simulink model "simz"  (R2018b)
settings: Solver=VariableStepAuto  StartTime=0.0  StopTime=500  RelTol=1e-3
undefined symbols (not defined in the file or in its folder): fswParams, MEKF_lib, test_lib
libraries: dspmtrx3 x2, sharedutil x2, aerolibutil x2, MEKF_Conversion_lib x1, Environment_lib x1, MEKF_lib x1, Sensors_Lib x1, satelliteDynamics_lib x1
settings Model: Creator=kylle  LastModifiedBy=kylle
settings DataIOCC: SaveFormat=StructureWithTime
settings DebuggingCC: SignalResolutionControl=None

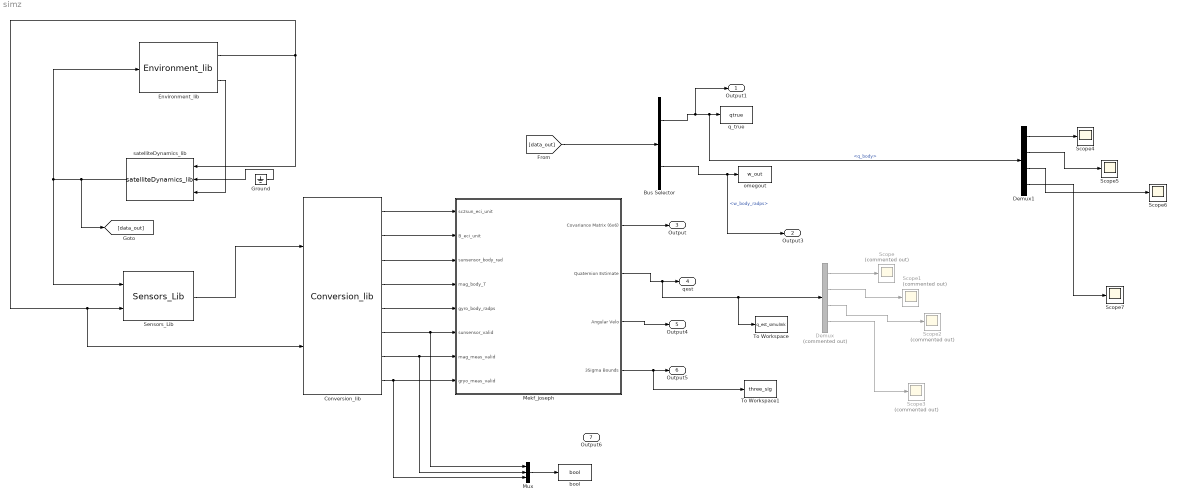
== system simz ==
  Bus Selector : BusSelector  OutputSignals=q_body,w_body_radps
  Conversion_lib : MEKF_Conversion_lib/Conversion_lib  SystemSampleTime=-1
  Demux : Demux  Commented=on
  Demux1 : Demux
  Environment_lib : Environment_lib/Environment_lib  SystemSampleTime=-1
  Ground : Ground
  Mekf_joseph : Subsystem  AncestorBlock=test_lib/MEKF_lib
  Mux : Mux  Inputs=3
  Scope{,1..3} (4 alike) : Scope  Commented=on
  Scope{4..7} (4 alike) : Scope
  Sensors_Lib : Sensors_Lib/Sensors_Lib  SystemSampleTime=-1
  To Workspace : ToWorkspace  VariableName=q_est_simulink  SaveFormat=Timeseries  SampleTime=-1
  To Workspace1 : ToWorkspace  VariableName=three_sig  SaveFormat=Timeseries  SampleTime=-1
  "bool " : ToWorkspace  VariableName=bool  SaveFormat=Timeseries  SampleTime=-1
  omegout : ToWorkspace  VariableName=w_out  SaveFormat=Timeseries  SampleTime=-1
  q_true : ToWorkspace  VariableName=qtrue  SaveFormat=Timeseries  SampleTime=-1
  satelliteDynamics_lib : satelliteDynamics_lib/satelliteDynamics_lib  SystemSampleTime=-1
  Output1 : Outport
  Output3 : Outport  Port=2
  Output : Outport  Port=3
  qest : Outport  Port=4
  Output4 : Outport  Port=5
  Output5 : Outport  Port=6
  Output6 : Outport  Port=7
  wires:
  satelliteDynamics_lib/1 -> [data_out], Environment_lib/1, Sensors_Lib/1
  Conversion_lib/2 -> Mekf_joseph/2(B_eci_unit)
  Conversion_lib/3 -> Mekf_joseph/3(sunsensor_body_rad)
  Conversion_lib/1 -> Mekf_joseph/1(sc2sun_eci_unit)
  Conversion_lib/4 -> Mekf_joseph/4(mag_body_T)
  Conversion_lib/5 -> Mekf_joseph/5(gyro_body_radps)
  Conversion_lib/6 -> Mux/1, Mekf_joseph/6(sunsensor_valid)
  Conversion_lib/7 -> Mux/2, Mekf_joseph/7(mag_meas_valid)
  Sensors_Lib/1 -> Conversion_lib/1
  Environment_lib/1 -> Conversion_lib/2, Sensors_Lib/2, satelliteDynamics_lib/1
  Ground/1 -> satelliteDynamics_lib/2
  Environment_lib/2 -> satelliteDynamics_lib/3
  Bus Selector/2 -> Output3/1, omegout/1  "<w_body_radps>"
  Bus Selector/1 -> Output1/1, Demux1/1, q_true/1  "<q_body>"
  [data_out] -> Bus Selector/1
  Mekf_joseph/1(Covariance Matrix (6x6)) -> Output/1
  Mekf_joseph/2("Quaternion Estimate ") -> To Workspace/1, Demux/1, qest/1
  Mekf_joseph/3("Angular Velo ") -> Output4/1
  Mekf_joseph/4("3Sigma Bounds ") -> To Workspace1/1, Output5/1
  Demux/1 -> Scope/1
  Demux/2 -> Scope1/1
  Demux/3 -> Scope2/1
  Demux/4 -> Scope3/1
  Demux1/1 -> Scope4/1
  Demux1/2 -> Scope5/1
  Demux1/4 -> Scope7/1
  Demux1/3 -> Scope6/1
  Conversion_lib/8 -> Mux/3, Mekf_joseph/8(gryo_meas_valid)
  Mux/1 -> "bool "/1

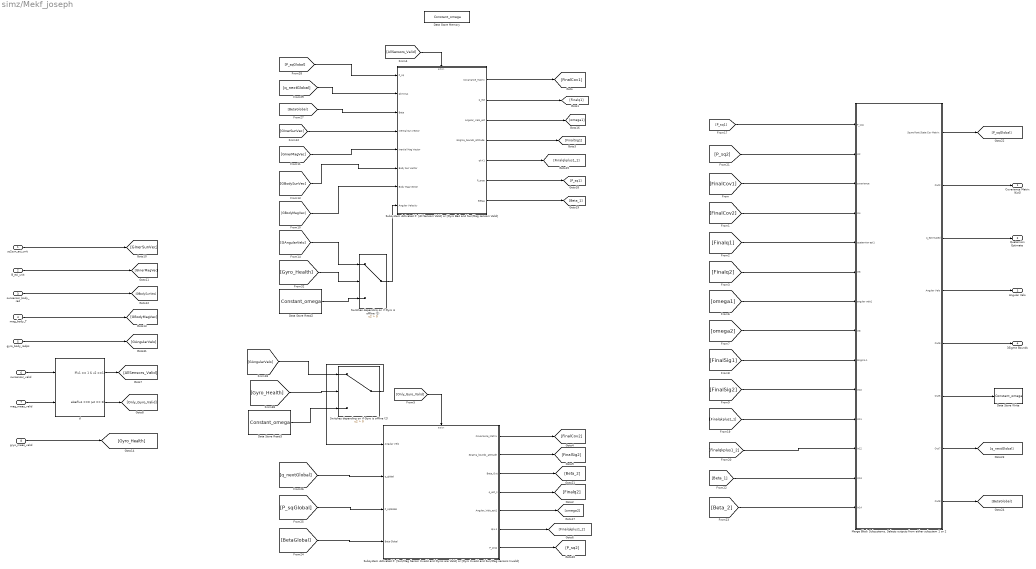
== system simz/Mekf_joseph ==
  sc2sun_eci_unit : Inport
  B_eci_unit : Inport  Port=2
  sunsensor_body_rad : Inport  Port=3
  mag_body_T : Inport  Port=4
  gyro_body_radps : Inport  Port=5
  sunsensor_valid : Inport  Port=6
  mag_meas_valid : Inport  Port=7
  gryo_meas_valid : Inport  Port=8
  Data Store Memory : DataStoreMemory  DataStoreName=Constant_omega  ReadBeforeWriteMsg=warning  WriteAfterWriteMsg=warning  WriteAfterReadMsg=warning  InitialValue=simParams.initialConditions.w0  VectorParams1D=off  ShowAdditionalParam=off
  Data Store Read2 : DataStoreRead  DataStoreName=Constant_omega
  Data Store Read3 : DataStoreRead  DataStoreName=Constant_omega
  Data Store Write : DataStoreWrite  DataStoreName=Constant_omega
  If : If  NumInputs=2  IfExpression=u1 == 1 & u2 ==1  ElseIfExpressions=u1 ==0 |u2 == 0  ShowElse=off
  "Merge Block Subsystems, Selects outputs from either subsytem 1 or 2" : Subsystem
  Subsystem Activated if: [All Sensors Valid] or [Gyro Bad and Sun/Mag sensors Valid] : Subsystem  TreatAsAtomicUnit=on
  Subsystem Activated if: [Sun/Mag Sensor Invalid and Gyros are Valid] or [Gyro Invalid and Sun/Mag sensors Invalid] : Subsystem  TreatAsAtomicUnit=on
  Switches depending on if Gyro is offline (1) : Switch  Criteria=u2 > Threshold
  Switches depending on if Gyro is offline (2) : Switch  Criteria=u2 > Threshold
  Covariance Matrix (6x6) : Outport
  "Quaternion Estimate " : Outport  Port=2
  "Angular Velo " : Outport  Port=3
  "3Sigma Bounds " : Outport  Port=4
  wires:
  gyro_body_radps/1 -> [GAngularVelo]
  mag_body_T/1 -> [GBodyMagVec]
  B_eci_unit/1 -> [GInerMagVec]
  gryo_meas_valid/1 -> [Gyro_Health]
  mag_meas_valid/1 -> If/2
  sunsensor_valid/1 -> If/1
  sunsensor_body_rad/1 -> [GBodySunVec]
  sc2sun_eci_unit/1 -> [GInerSunVec]
  "Merge Block Subsystems, Selects outputs from either subsytem 1 or 2"/8(Out8) -> [BetaGlobal]
  "Merge Block Subsystems, Selects outputs from either subsytem 1 or 2"/7(Out7) -> [q_nextGlobal]
  "Merge Block Subsystems, Selects outputs from either subsytem 1 or 2"/5(Out6) -> "3Sigma Bounds "/1
  "Merge Block Subsystems, Selects outputs from either subsytem 1 or 2"/6(Out5) -> Data Store Write/1
  "Merge Block Subsystems, Selects outputs from either subsytem 1 or 2"/4(Angular Velo) -> "Angular Velo "/1
  "Merge Block Subsystems, Selects outputs from either subsytem 1 or 2"/3(q_estimated) -> "Quaternion Estimate "/1
  "Merge Block Subsystems, Selects outputs from either subsytem 1 or 2"/2(Out2) -> Covariance Matrix (6x6)/1
  "Merge Block Subsystems, Selects outputs from either subsytem 1 or 2"/1(Squre Root State Cov Matrix) -> [P_sqGlobal]
  [Beta_2] -> "Merge Block Subsystems, Selects outputs from either subsytem 1 or 2"/14(In14)
  [Beta_1] -> "Merge Block Subsystems, Selects outputs from either subsytem 1 or 2"/13(In13)
  [Finalqkplus1_2] -> "Merge Block Subsystems, Selects outputs from either subsytem 1 or 2"/12(In12)
  [Finalqkplus1_1] -> "Merge Block Subsystems, Selects outputs from either subsytem 1 or 2"/11(In11)
  [FinalSig2] -> "Merge Block Subsystems, Selects outputs from either subsytem 1 or 2"/10(In10)
  [FinalSig1] -> "Merge Block Subsystems, Selects outputs from either subsytem 1 or 2"/9(3sigma 1)
  [omega2] -> "Merge Block Subsystems, Selects outputs from either subsytem 1 or 2"/8(In8)
  [omega1] -> "Merge Block Subsystems, Selects outputs from either subsytem 1 or 2"/7(angular velo1)
  [Finalq2] -> "Merge Block Subsystems, Selects outputs from either subsytem 1 or 2"/6(In6)
  [Finalq1] -> "Merge Block Subsystems, Selects outputs from either subsytem 1 or 2"/5(quaternion est1)
  [FinalCov2] -> "Merge Block Subsystems, Selects outputs from either subsytem 1 or 2"/4(In4)
  [FinalCov1] -> "Merge Block Subsystems, Selects outputs from either subsytem 1 or 2"/3(covariance)
  [P_sq2] -> "Merge Block Subsystems, Selects outputs from either subsytem 1 or 2"/2(In2)
  [P_sq1] -> "Merge Block Subsystems, Selects outputs from either subsytem 1 or 2"/1(P_sq1)
  Data Store Read3/1 -> Switches depending on if Gyro is offline (2)/3
  [Gyro_Health] -> Switches depending on if Gyro is offline (2)/2
  Data Store Read2/1 -> Switches depending on if Gyro is offline (1)/3
  [Gyro_Health] -> Switches depending on if Gyro is offline (1)/2
  If/2 -> [Only_Gyro_Valid]
  If/1 -> [AllSensors_Valid]
  [P_sqGlobal] -> Subsystem Activated if: [All Sensors Valid] or [Gyro Bad and Sun/Mag sensors Valid]/1(P_sq)
  [q_nextGlobal] -> Subsystem Activated if: [All Sensors Valid] or [Gyro Bad and Sun/Mag sensors Valid]/2(qkminus)
  Subsystem Activated if: [Sun/Mag Sensor Invalid and Gyros are Valid] or [Gyro Invalid and Sun/Mag sensors Invalid]/5(Angular_Velo_est1) -> [omega2]
  Subsystem Activated if: [Sun/Mag Sensor Invalid and Gyros are Valid] or [Gyro Invalid and Sun/Mag sensors Invalid]/3(Beta_Out) -> [Beta_2]
  Subsystem Activated if: [Sun/Mag Sensor Invalid and Gyros are Valid] or [Gyro Invalid and Sun/Mag sensors Invalid]/7("P_prop ") -> [P_sq2]
  Subsystem Activated if: [All Sensors Valid] or [Gyro Bad and Sun/Mag sensors Valid]/7(Betaa) -> [Beta_1]
  Subsystem Activated if: [All Sensors Valid] or [Gyro Bad and Sun/Mag sensors Valid]/6("P_prop ") -> [P_sq1]
  Subsystem Activated if: [All Sensors Valid] or [Gyro Bad and Sun/Mag sensors Valid]/3(Angular_Velo_est) -> [omega1]
  [BetaGlobal] -> Subsystem Activated if: [All Sensors Valid] or [Gyro Bad and Sun/Mag sensors Valid]/3(Beta)
  [BetaGlobal] -> Subsystem Activated if: [Sun/Mag Sensor Invalid and Gyros are Valid] or [Gyro Invalid and Sun/Mag sensors Invalid]/4(Beta Global)
  [P_sqGlobal] -> Subsystem Activated if: [Sun/Mag Sensor Invalid and Gyros are Valid] or [Gyro Invalid and Sun/Mag sensors Invalid]/3(P_sqGlobal)
  Subsystem Activated if: [All Sensors Valid] or [Gyro Bad and Sun/Mag sensors Valid]/5(qk+1) -> [Finalqkplus1_1]
  [q_nextGlobal] -> Subsystem Activated if: [Sun/Mag Sensor Invalid and Gyros are Valid] or [Gyro Invalid and Sun/Mag sensors Invalid]/2(q_global)
  Subsystem Activated if: [Sun/Mag Sensor Invalid and Gyros are Valid] or [Gyro Invalid and Sun/Mag sensors Invalid]/2(3sigma_bounds_attitude) -> [FinalSig2]
  [AllSensors_Valid] -> Subsystem Activated if: [All Sensors Valid] or [Gyro Bad and Sun/Mag sensors Valid]/Action
  Subsystem Activated if: [Sun/Mag Sensor Invalid and Gyros are Valid] or [Gyro Invalid and Sun/Mag sensors Invalid]/1(Covariance_Matrix) -> [FinalCov2]
  [GInerSunVec] -> Subsystem Activated if: [All Sensors Valid] or [Gyro Bad and Sun/Mag sensors Valid]/4(Inertial Sun Vector)
  Subsystem Activated if: [Sun/Mag Sensor Invalid and Gyros are Valid] or [Gyro Invalid and Sun/Mag sensors Invalid]/4(q_est_k) -> [Finalq2]
  Subsystem Activated if: [All Sensors Valid] or [Gyro Bad and Sun/Mag sensors Valid]/4(3sigma_bounds_attitude) -> [FinalSig1]
  [Only_Gyro_Valid] -> Subsystem Activated if: [Sun/Mag Sensor Invalid and Gyros are Valid] or [Gyro Invalid and Sun/Mag sensors Invalid]/Action
  Subsystem Activated if: [All Sensors Valid] or [Gyro Bad and Sun/Mag sensors Valid]/1(Covariance_Matrix) -> [FinalCov1]
  [GBodyMagVec] -> Subsystem Activated if: [All Sensors Valid] or [Gyro Bad and Sun/Mag sensors Valid]/7(Body Mag Vector)
  [GInerMagVec] -> Subsystem Activated if: [All Sensors Valid] or [Gyro Bad and Sun/Mag sensors Valid]/5(Inertial Mag Vector)
  [GBodySunVec] -> Subsystem Activated if: [All Sensors Valid] or [Gyro Bad and Sun/Mag sensors Valid]/6(Body Sun Vector)
  [GAngularVelo] -> Switches depending on if Gyro is offline (2)/1
  [GAngularVelo] -> Switches depending on if Gyro is offline (1)/1
  Switches depending on if Gyro is offline (1)/1 -> Subsystem Activated if: [All Sensors Valid] or [Gyro Bad and Sun/Mag sensors Valid]/8(Angular Velocity)
  Switches depending on if Gyro is offline (2)/1 -> Subsystem Activated if: [Sun/Mag Sensor Invalid and Gyros are Valid] or [Gyro Invalid and Sun/Mag sensors Invalid]/1(Angular Velo)
  Subsystem Activated if: [Sun/Mag Sensor Invalid and Gyros are Valid] or [Gyro Invalid and Sun/Mag sensors Invalid]/6(qk+1) -> [Finalqkplus1_2]
  Subsystem Activated if: [All Sensors Valid] or [Gyro Bad and Sun/Mag sensors Valid]/2(q_est) -> [Finalq1]

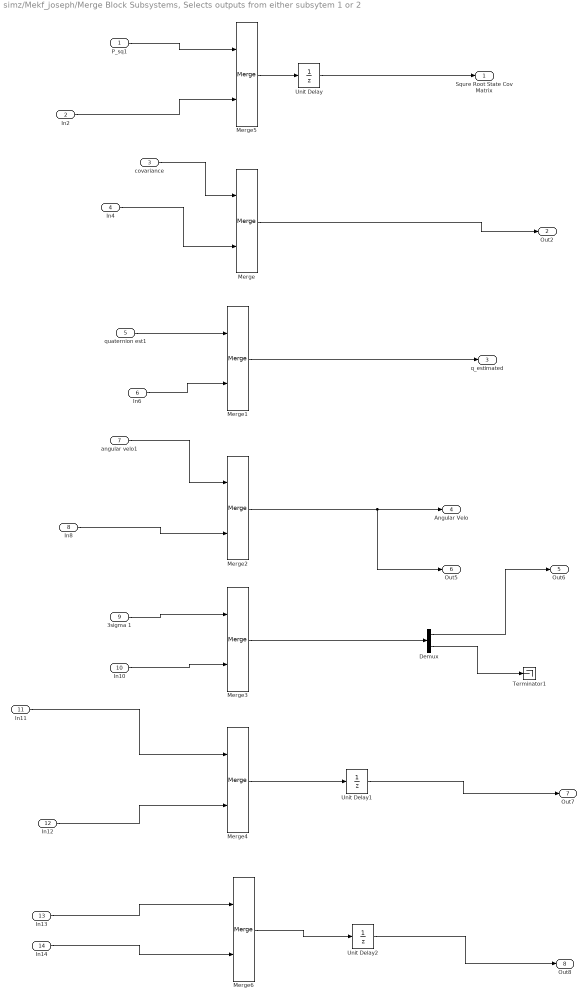
== system simz/Mekf_joseph/Merge Block Subsystems, Selects outputs from either subsytem 1 or 2 ==
  P_sq1 : Inport
  In2 : Inport  Port=2
  covariance : Inport  Port=3
  In4 : Inport  Port=4
  quaternion est1 : Inport  Port=5
  In6 : Inport  Port=6
  angular velo1 : Inport  Port=7
  In8 : Inport  Port=8
  3sigma 1 : Inport  Port=9
  In10 : Inport  Port=10
  In11 : Inport  Port=11
  In12 : Inport  Port=12
  In13 : Inport  Port=13
  In14 : Inport  Port=14
  Demux : Demux  Outputs=2
  Merge{,1..6} (7 alike) : Merge
  Terminator1 : Terminator
  Unit Delay : UnitDelay  InitialCondition=fswParams.estimation.ic.P_init  SampleTime=-1
  Unit Delay1 : UnitDelay  InitialCondition=fswParams.estimation.ic.quat_est_init  SampleTime=-1
  Unit Delay2 : UnitDelay  InitialCondition=fswParams.estimation.ic.Beta_init  SampleTime=-1
  Squre Root State Cov Matrix : Outport
  Out2 : Outport  Port=2
  q_estimated : Outport  Port=3
  Angular Velo : Outport  Port=4
  Out6 : Outport  Port=5
  Out5 : Outport  Port=6
  Out7 : Outport  Port=7
  Out8 : Outport  Port=8
  wires:
  Merge1/1 -> q_estimated/1
  Unit Delay/1 -> Squre Root State Cov Matrix/1
  Unit Delay2/1 -> Out8/1
  P_sq1/1 -> Merge5/1
  In12/1 -> Merge4/2
  In8/1 -> Merge2/2
  In6/1 -> Merge1/2
  Merge/1 -> Out2/1
  In13/1 -> Merge6/1
  Demux/1 -> Out6/1
  In4/1 -> Merge/2
  Merge4/1 -> Unit Delay1/1
  covariance/1 -> Merge/1
  In2/1 -> Merge5/2
  In10/1 -> Merge3/2
  Merge5/1 -> Unit Delay/1
  In11/1 -> Merge4/1
  angular velo1/1 -> Merge2/1
  In14/1 -> Merge6/2
  quaternion est1/1 -> Merge1/1
  3sigma 1/1 -> Merge3/1
  Merge6/1 -> Unit Delay2/1
  Demux/2 -> Terminator1/1
  Unit Delay1/1 -> Out7/1
  Merge2/1 -> Angular Velo/1, Out5/1
  Merge3/1 -> Demux/1

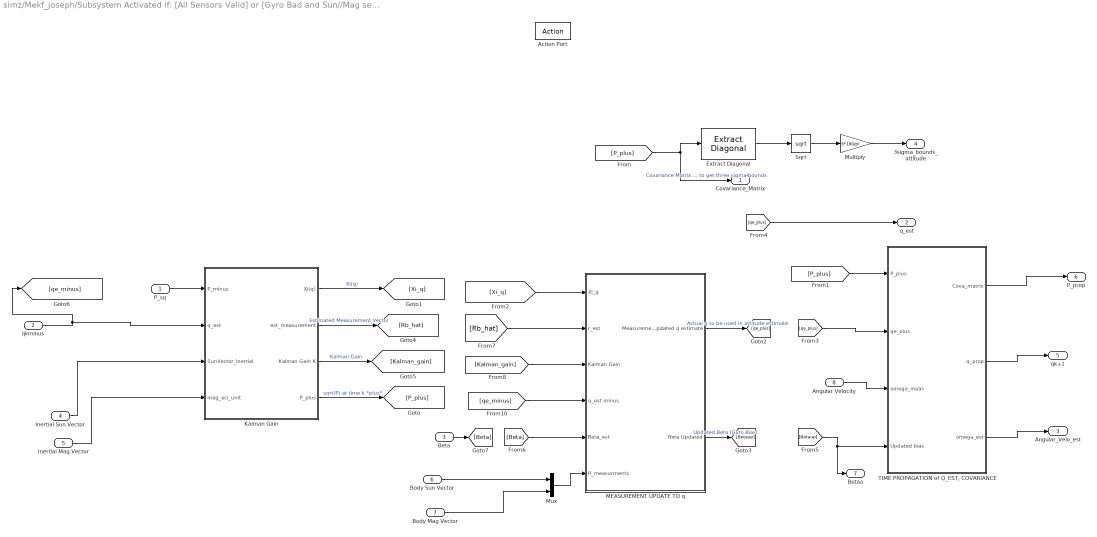
== system simz/Mekf_joseph/Subsystem Activated if: [All Sensors Valid] or [Gyro Bad and Sun//Mag sensors Valid] ==
  P_sq : Inport
  qkminus : Inport  Port=2
  Beta : Inport  Port=3
  Inertial Sun Vector : Inport  Port=4
  Inertial Mag Vector : Inport  Port=5
  Body Sun Vector : Inport  Port=6
  Body Mag Vector : Inport  Port=7
  Angular Velocity : Inport  Port=8
  Action Port : ActionPort  ActionType=then
  Extract Diagonal : dspmtrx3/Extract Diagonal
      settings: SourceProductName=DSP System Toolbox  SourceProductBaseCode=DS
  Kalman Gain : Subsystem  AncestorBlock=MEKF_LibraryR2018b/Multiplicative Extended Kalman Filter/Kalman Gain
  "MEASUREMENT UPDATE TO q " : Subsystem  AncestorBlock=MEKF_LibraryR2018b/Multiplicative Extended Kalman Filter/MEASUREMENT UPDATE TO q AND COVARIANCE2
  Multiply : Gain  Gain=3*180/pi
  Mux : Mux  Inputs=2
  Sqrt : Sqrt  SaturateOnIntegerOverflow=on
  "TIME PROPAGATION of Q_EST, COVARIANCE" : Subsystem  AncestorBlock=MEKF_Library/Multiplicative Extended Kalman Filter/TIME PROPAGATION of Q_EST, COVARIANCE
  Covariance_Matrix : Outport
  q_est : Outport  Port=2
  Angular_Velo_est : Outport  Port=3
  3sigma_bounds_attitude : Outport  Port=4
  qk+1 : Outport  Port=5
  "P_prop " : Outport  Port=6
  Betaa : Outport  Port=7
  wires:
  Beta/1 -> [Beta]
  Multiply/1 -> 3sigma_bounds_attitude/1
  Mux/1 -> "MEASUREMENT UPDATE TO q "/6(R_measurments)
  Body Mag Vector/1 -> Mux/2
  Body Sun Vector/1 -> Mux/1
  Inertial Mag Vector/1 -> Kalman Gain/4("mag_eci_unit ")
  [Kalman_gain] -> "MEASUREMENT UPDATE TO q "/3(Kalman Gain)
  [Xi_q] -> "MEASUREMENT UPDATE TO q "/1(Xi_q)
  Kalman Gain/2(est_measurement) -> [Rb_hat]  "Estimated Measurement Vector"
  [P_plus] -> "TIME PROPAGATION of Q_EST, COVARIANCE"/1(P_plus)
  "MEASUREMENT UPDATE TO q "/1(Measurement updated q estimate) -> [qe_plus]  "Actual q to be used in attitude estimate"
  [Beta] -> "MEASUREMENT UPDATE TO q "/5(Beta_est)
  [Betaup] -> Betaa/1, "TIME PROPAGATION of Q_EST, COVARIANCE"/4(Updated bias)
  Sqrt/1 -> Multiply/1
  Kalman Gain/1(Xi(q)) -> [Xi_q]  "Xi(q)"
  [qe_minus] -> "MEASUREMENT UPDATE TO q "/4(q_est minus)
  Kalman Gain/3(Kalman Gain K) -> [Kalman_gain]  "Kalman Gain"
  Kalman Gain/4(P_plus) -> [P_plus]  "sqrt(P) at time k *plus*"
  "TIME PROPAGATION of Q_EST, COVARIANCE"/1(Cova_matrix) -> "P_prop "/1
  [Rb_hat] -> "MEASUREMENT UPDATE TO q "/2(r_est)
  "MEASUREMENT UPDATE TO q "/2(Beta Updated) -> [Betaup]  "Updated Beta (Gyro Bias)"
  [qe_plus] -> "TIME PROPAGATION of Q_EST, COVARIANCE"/2(qe_plus)
  P_sq/1 -> Kalman Gain/1(P_minus)
  Angular Velocity/1 -> "TIME PROPAGATION of Q_EST, COVARIANCE"/3(omega_meas)
  Extract Diagonal/1 -> Sqrt/1
  qkminus/1 -> Kalman Gain/2(q_est), [qe_minus]
  [P_plus] -> Covariance_Matrix/1, Extract Diagonal/1  "Covariance Matrix from which to get three sigma bounds"
  "TIME PROPAGATION of Q_EST, COVARIANCE"/3(omega_est) -> Angular_Velo_est/1
  "TIME PROPAGATION of Q_EST, COVARIANCE"/2(q_prop) -> qk+1/1
  Inertial Sun Vector/1 -> Kalman Gain/3(SunVector_Inertial)
  [qe_plus] -> q_est/1

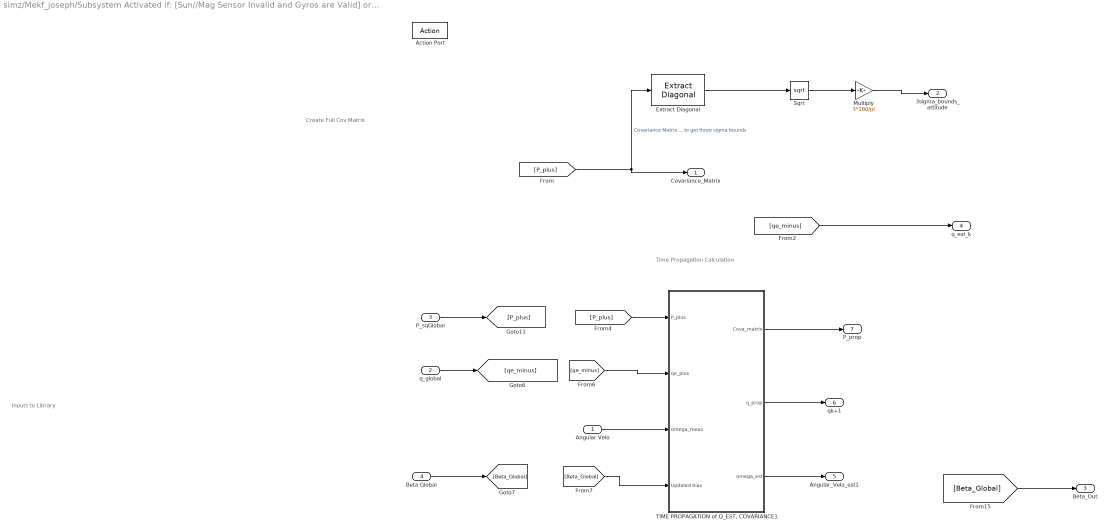
== system simz/Mekf_joseph/Subsystem Activated if: [Sun//Mag Sensor Invalid and Gyros are Valid] or [Gyro Invalid and Sun//Mag sensors Invalid] ==
  note: Create Full Cov Matrix
  note: Inputs to Library
  note: Time Propagation Calculation
  Angular Velo : Inport
  q_global : Inport  Port=2
  P_sqGlobal : Inport  Port=3
  Beta Global : Inport  Port=4
  Action Port : ActionPort  ActionType=elseif
  Extract Diagonal : dspmtrx3/Extract Diagonal
      settings: SourceProductName=DSP System Toolbox  SourceProductBaseCode=DS
  Multiply : Gain  Gain=3*180/pi
  Sqrt : Sqrt  SaturateOnIntegerOverflow=on
  "TIME PROPAGATION of Q_EST, COVARIANCE1" : Subsystem  AncestorBlock=MEKF_Library/Multiplicative Extended Kalman Filter/TIME PROPAGATION of Q_EST, COVARIANCE
  Covariance_Matrix : Outport
  3sigma_bounds_attitude : Outport  Port=2
  Beta_Out : Outport  Port=3
  q_est_k : Outport  Port=4
  Angular_Velo_est1 : Outport  Port=5
  qk+1 : Outport  Port=6
  "P_prop " : Outport  Port=7
  wires:
  Sqrt/1 -> Multiply/1
  Multiply/1 -> 3sigma_bounds_attitude/1
  [Beta_Global] -> Beta_Out/1
  [P_plus] -> Covariance_Matrix/1, Extract Diagonal/1  "Covariance Matrix from which to get three sigma bounds"
  [qe_minus] -> q_est_k/1
  P_sqGlobal/1 -> [P_plus]
  Extract Diagonal/1 -> Sqrt/1
  Beta Global/1 -> [Beta_Global]
  q_global/1 -> [qe_minus]
  [qe_minus] -> "TIME PROPAGATION of Q_EST, COVARIANCE1"/2(qe_plus)
  Angular Velo/1 -> "TIME PROPAGATION of Q_EST, COVARIANCE1"/3(omega_meas)
  "TIME PROPAGATION of Q_EST, COVARIANCE1"/3(omega_est) -> Angular_Velo_est1/1
  [Beta_Global] -> "TIME PROPAGATION of Q_EST, COVARIANCE1"/4(Updated bias)
  "TIME PROPAGATION of Q_EST, COVARIANCE1"/1(Cova_matrix) -> "P_prop "/1
  "TIME PROPAGATION of Q_EST, COVARIANCE1"/2(q_prop) -> qk+1/1
  [P_plus] -> "TIME PROPAGATION of Q_EST, COVARIANCE1"/1(P_plus)

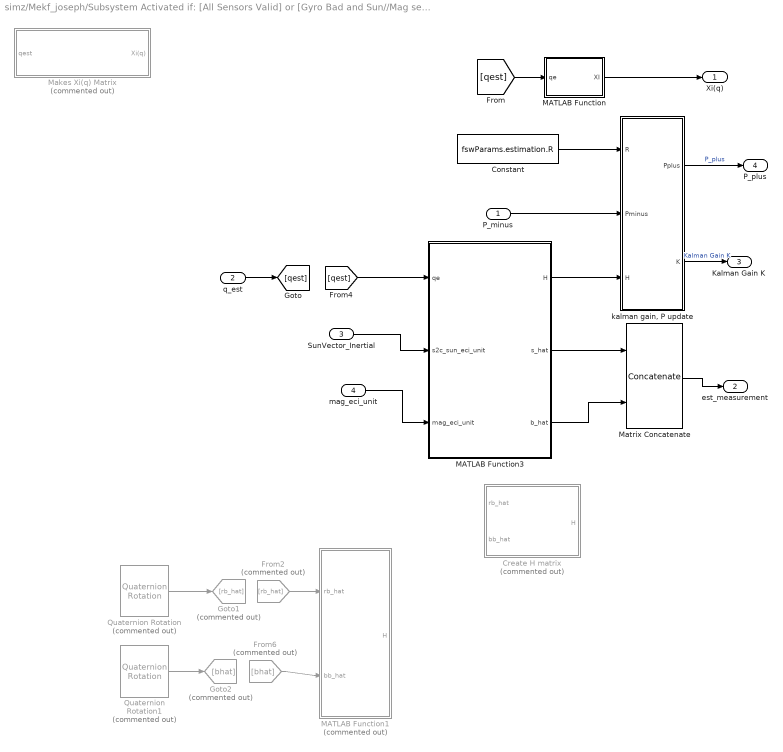
== system simz/Mekf_joseph/Subsystem Activated if: [All Sensors Valid] or [Gyro Bad and Sun//Mag sensors Valid]/Kalman Gain ==
  P_minus : Inport
  q_est : Inport  Port=2
  SunVector_Inertial : Inport  Port=3
  "mag_eci_unit " : Inport  Port=4
  Constant : Constant  Value=fswParams.estimation.R  VectorParams1D=off
  Create H matrix : Subsystem  Commented=on
  From2 : From  Commented=on  GotoTag=rb_hat
  From6 : From  Commented=on  GotoTag=bhat
  Goto1 : Goto  Commented=on  GotoTag=rb_hat
  Goto2 : Goto  Commented=on  GotoTag=bhat
  MATLAB Function : MATLAB Function  TreatAsAtomicUnit=on
  MATLAB Function1 : MATLAB Function  Commented=on  TreatAsAtomicUnit=on
  MATLAB Function3 : MATLAB Function  TreatAsAtomicUnit=on
  Makes Xi(q) Matrix : Subsystem  Commented=on
  Matrix Concatenate : Concatenate  Mode=Multidimensional array
  Quaternion Rotation : aerolibutil/Quaternion Rotation  Commented=on
  Quaternion Rotation1 : aerolibutil/Quaternion Rotation  Commented=on
  "kalman gain, P update" : MATLAB Function  TreatAsAtomicUnit=on
  Xi(q) : Outport
  est_measurement : Outport  Port=2
  Kalman Gain K : Outport  Port=3
  P_plus : Outport  Port=4
  wires:
  MATLAB Function/1(XI) -> Xi(q)/1
  [qest] -> MATLAB Function/1(qe)
  Constant/1 -> "kalman gain, P update"/1(R)
  Matrix Concatenate/1 -> est_measurement/1
  MATLAB Function3/3(b_hat) -> Matrix Concatenate/2
  MATLAB Function3/2(s_hat) -> Matrix Concatenate/1
  Quaternion Rotation1/1 -> Goto2/1
  Quaternion Rotation/1 -> Goto1/1
  q_est/1 -> [qest]
  "kalman gain, P update"/1(Pplus) -> P_plus/1  "P_plus"
  "kalman gain, P update"/2(K) -> Kalman Gain K/1  "Kalman Gain K"
  P_minus/1 -> "kalman gain, P update"/2(Pminus)
  From2/1 -> MATLAB Function1/1(rb_hat)
  From6/1 -> MATLAB Function1/2(bb_hat)
  [qest] -> MATLAB Function3/1(qe)
  SunVector_Inertial/1 -> MATLAB Function3/2(s2c_sun_eci_unit)
  "mag_eci_unit "/1 -> MATLAB Function3/3(mag_eci_unit)
  MATLAB Function3/1(H) -> "kalman gain, P update"/3(H)

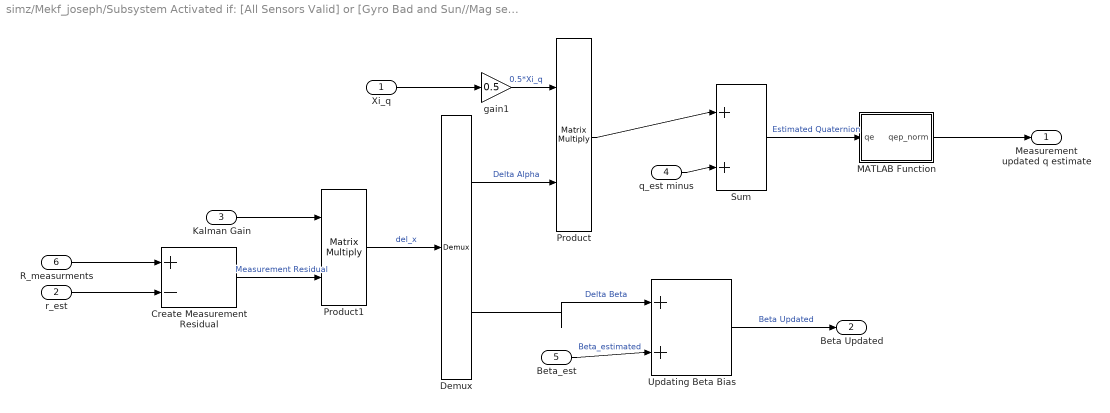
== system simz/Mekf_joseph/Subsystem Activated if: [All Sensors Valid] or [Gyro Bad and Sun//Mag sensors Valid]/MEASUREMENT UPDATE TO q  ==
  Xi_q : Inport
  r_est : Inport  Port=2
  Kalman Gain : Inport  Port=3
  q_est minus : Inport  Port=4
  Beta_est : Inport  Port=5
  R_measurments : Inport  Port=6
  Create Measurement Residual : Sum  Inputs=+-
  Demux : Demux  Outputs=2
  MATLAB Function : MATLAB Function  TreatAsAtomicUnit=on
  Product : Product  Inputs=**  Multiplication=Matrix(*)
  Product1 : Product  Multiplication=Matrix(*)
  Sum : Sum  Inputs=|++
  "Updating Beta Bias " : Sum  Inputs=|++
  gain1 : Gain  Gain=0.5
  Measurement updated q estimate : Outport
  Beta Updated : Outport  Port=2
  wires:
  MATLAB Function/1(qep_norm) -> Measurement updated q estimate/1
  Sum/1 -> MATLAB Function/1(qe)  "Estimated Quaternion"
  Xi_q/1 -> gain1/1
  R_measurments/1 -> Create Measurement Residual/1
  Kalman Gain/1 -> Product1/1
  q_est minus/1 -> Sum/2
  Beta_est/1 -> "Updating Beta Bias "/2  "Beta_estimated"
  "Updating Beta Bias "/1 -> Beta Updated/1  "Beta Updated"
  Create Measurement Residual/1 -> Product1/2  "Measurement Residual"
  r_est/1 -> Create Measurement Residual/2
  Product1/1 -> Demux/1  "del_x"
  Product/1 -> Sum/1
  Demux/2 -> "Updating Beta Bias "/1  "Delta Beta"
  gain1/1 -> Product/1  "0.5*Xi_q"
  Demux/1 -> Product/2  "Delta Alpha"

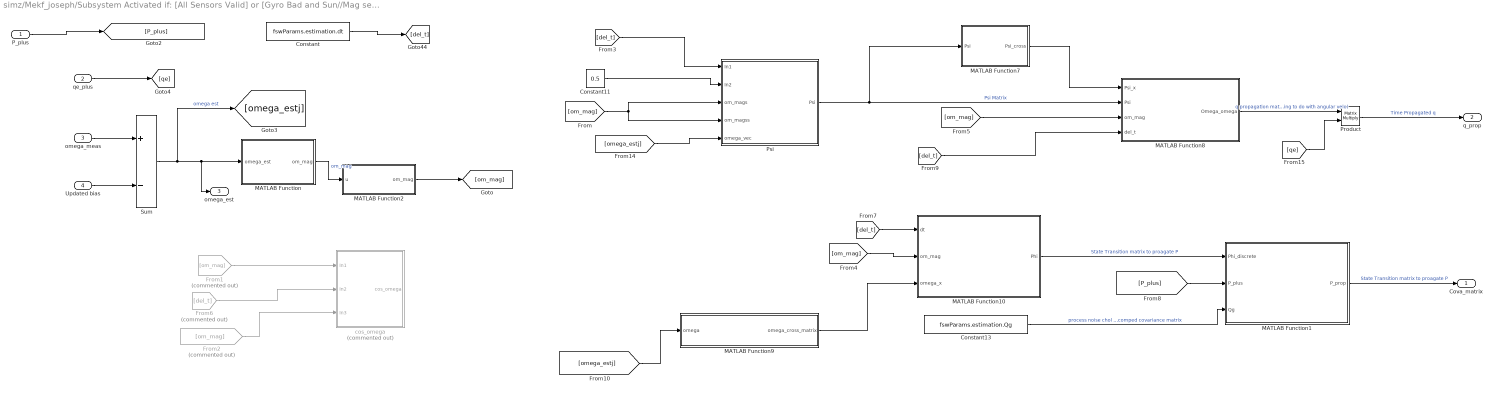
== system simz/Mekf_joseph/Subsystem Activated if: [All Sensors Valid] or [Gyro Bad and Sun//Mag sensors Valid]/TIME PROPAGATION of Q_EST, COVARIANCE ==
  P_plus : Inport
  qe_plus : Inport  Port=2
  omega_meas : Inport  Port=3
  Updated bias : Inport  Port=4
  Constant : Constant  Value=fswParams.estimation.dt
  Constant11 : Constant  Value=0.5
  Constant13 : Constant  Value=fswParams.estimation.Qg  VectorParams1D=off
  From1 : From  Commented=on  GotoTag=om_mag
  From2 : From  Commented=on  GotoTag=om_mag
  From6 : From  Commented=on  GotoTag=del_t
  MATLAB Function : MATLAB Function  TreatAsAtomicUnit=on
  MATLAB Function1 : MATLAB Function  TreatAsAtomicUnit=on
  MATLAB Function10 : MATLAB Function  TreatAsAtomicUnit=on
  MATLAB Function2 : MATLAB Function  TreatAsAtomicUnit=on
  MATLAB Function7 : MATLAB Function  TreatAsAtomicUnit=on
  MATLAB Function8 : MATLAB Function  TreatAsAtomicUnit=on
  MATLAB Function9 : MATLAB Function  TreatAsAtomicUnit=on
  Product : Product  Multiplication=Matrix(*)
  Psi : Subsystem
  Sum : Sum  Inputs=+-
  cos_omega : Subsystem  Commented=on
  Cova_matrix : Outport
  q_prop : Outport  Port=2
  omega_est : Outport  Port=3
  wires:
  MATLAB Function1/1(P_prop) -> Cova_matrix/1  "State Transition matrix to proagate P"
  MATLAB Function2/1(om_mag) -> [om_mag]
  Constant/1 -> [del_t]
  From6/1 -> cos_omega/2(In2)
  Sum/1 -> [omega_estj], omega_est/1, MATLAB Function/1(omega_est)  "omega est"
  [om_mag] -> Psi/4(om_magss), Psi/3(om_mags)
  [omega_estj] -> Psi/5(omega_vec)
  Constant11/1 -> Psi/2(In2)
  [del_t] -> Psi/1(In1)
  Psi/1(Psi) -> MATLAB Function7/1(Psi), MATLAB Function8/2(Psi)  "Psi Matrix"
  From2/1 -> cos_omega/3(In3)
  From1/1 -> cos_omega/1(In1)
  [qe] -> Product/2
  [omega_estj] -> MATLAB Function9/1(omega)
  [P_plus] -> MATLAB Function1/2(P_plus)
  [del_t] -> MATLAB Function10/1(dt)
  [om_mag] -> MATLAB Function8/3(om_mag)
  [om_mag] -> MATLAB Function10/2(om_mag)
  MATLAB Function/1(om_mag) -> MATLAB Function2/1(u)  "om_mag"
  Constant13/1 -> MATLAB Function1/3(Qg)  "process noise chol decomped covariance matrix"
  Product/1 -> q_prop/1  "Time Propagated q"
  MATLAB Function10/1(Phi) -> MATLAB Function1/1(Phi_discrete)  "State Transition matrix to proagate P"
  MATLAB Function9/1(omega_cross_matrix) -> MATLAB Function10/3(omega_x)
  MATLAB Function8/1(Omega_omega) -> Product/1  "q propagation matrix (nothing to do with angular velo)"
  MATLAB Function7/1(Psi_cross) -> MATLAB Function8/1(Psi_x)
  [del_t] -> MATLAB Function8/4(del_t)
  omega_meas/1 -> Sum/1
  Updated bias/1 -> Sum/2
  qe_plus/1 -> [qe]
  P_plus/1 -> [P_plus]

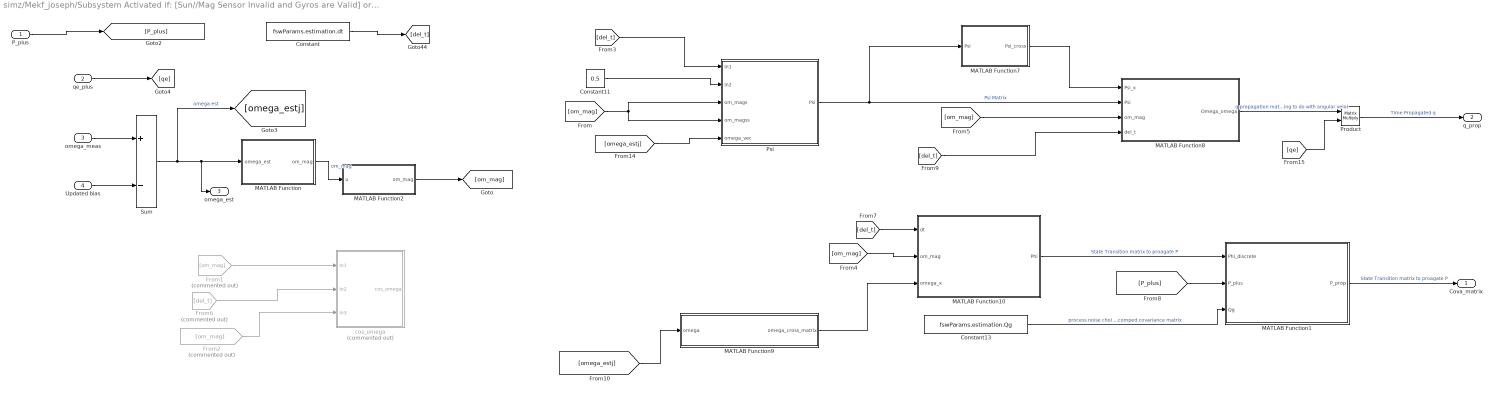
== system simz/Mekf_joseph/Subsystem Activated if: [Sun//Mag Sensor Invalid and Gyros are Valid] or [Gyro Invalid and Sun//Mag sensors Invalid]/TIME PROPAGATION of Q_EST, COVARIANCE1 ==
  P_plus : Inport
  qe_plus : Inport  Port=2
  omega_meas : Inport  Port=3
  Updated bias : Inport  Port=4
  Constant : Constant  Value=fswParams.estimation.dt
  Constant11 : Constant  Value=0.5
  Constant13 : Constant  Value=fswParams.estimation.Qg  VectorParams1D=off
  From1 : From  Commented=on  GotoTag=om_mag
  From2 : From  Commented=on  GotoTag=om_mag
  From6 : From  Commented=on  GotoTag=del_t
  MATLAB Function : MATLAB Function  TreatAsAtomicUnit=on
  MATLAB Function1 : MATLAB Function  TreatAsAtomicUnit=on
  MATLAB Function10 : MATLAB Function  TreatAsAtomicUnit=on
  MATLAB Function2 : MATLAB Function  TreatAsAtomicUnit=on
  MATLAB Function7 : MATLAB Function  TreatAsAtomicUnit=on
  MATLAB Function8 : MATLAB Function  TreatAsAtomicUnit=on
  MATLAB Function9 : MATLAB Function  TreatAsAtomicUnit=on
  Product : Product  Multiplication=Matrix(*)
  Psi : Subsystem
  Sum : Sum  Inputs=+-
  cos_omega : Subsystem  Commented=on
  Cova_matrix : Outport
  q_prop : Outport  Port=2
  omega_est : Outport  Port=3
  wires:
  MATLAB Function1/1(P_prop) -> Cova_matrix/1  "State Transition matrix to proagate P"
  MATLAB Function2/1(om_mag) -> [om_mag]
  Constant/1 -> [del_t]
  From6/1 -> cos_omega/2(In2)
  Sum/1 -> [omega_estj], omega_est/1, MATLAB Function/1(omega_est)  "omega est"
  [om_mag] -> Psi/4(om_magss), Psi/3(om_mags)
  [omega_estj] -> Psi/5(omega_vec)
  Constant11/1 -> Psi/2(In2)
  [del_t] -> Psi/1(In1)
  Psi/1(Psi) -> MATLAB Function7/1(Psi), MATLAB Function8/2(Psi)  "Psi Matrix"
  From2/1 -> cos_omega/3(In3)
  From1/1 -> cos_omega/1(In1)
  [qe] -> Product/2
  [omega_estj] -> MATLAB Function9/1(omega)
  [P_plus] -> MATLAB Function1/2(P_plus)
  [del_t] -> MATLAB Function10/1(dt)
  [om_mag] -> MATLAB Function8/3(om_mag)
  [om_mag] -> MATLAB Function10/2(om_mag)
  MATLAB Function/1(om_mag) -> MATLAB Function2/1(u)  "om_mag"
  Constant13/1 -> MATLAB Function1/3(Qg)  "process noise chol decomped covariance matrix"
  Product/1 -> q_prop/1  "Time Propagated q"
  MATLAB Function10/1(Phi) -> MATLAB Function1/1(Phi_discrete)  "State Transition matrix to proagate P"
  MATLAB Function9/1(omega_cross_matrix) -> MATLAB Function10/3(omega_x)
  MATLAB Function8/1(Omega_omega) -> Product/1  "q propagation matrix (nothing to do with angular velo)"
  MATLAB Function7/1(Psi_cross) -> MATLAB Function8/1(Psi_x)
  [del_t] -> MATLAB Function8/4(del_t)
  omega_meas/1 -> Sum/1
  Updated bias/1 -> Sum/2
  qe_plus/1 -> [qe]
  P_plus/1 -> [P_plus]

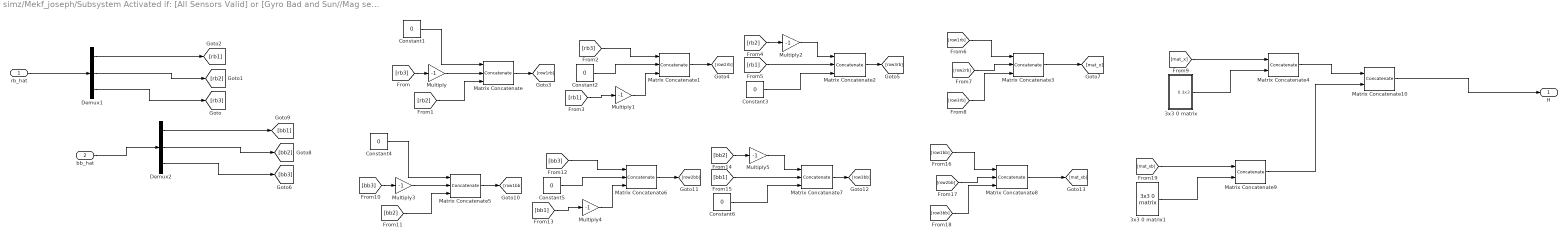
== system simz/Mekf_joseph/Subsystem Activated if: [All Sensors Valid] or [Gyro Bad and Sun//Mag sensors Valid]/Kalman Gain/Create H matrix ==
  rb_hat : Inport
  bb_hat : Inport  Port=2
  3x3 0 matrix : Subsystem
  3x3 0 matrix1 : MEKF_lib/MEKF_lib/Subsystem Activated if: [All Sensors Valid] or [Gyro Bad and Sun//Mag sensors Valid]/Kalman Gain/Create H matrix/3x3 0 matrix  SystemSampleTime=-1
  Constant{1..6} (6 alike) : Constant  Value=0
  Demux1 : Demux  Outputs=3
  Demux2 : Demux  Outputs=3
  Matrix Concatenate{,1..2,5..7} (6 alike) : Concatenate  NumInputs=3  Mode=Multidimensional array  ConcatenateDimension=2
  Matrix Concatenate10 : Concatenate  Mode=Multidimensional array
  Matrix Concatenate3 : Concatenate  NumInputs=3  Mode=Multidimensional array
  Matrix Concatenate4 : Concatenate  Mode=Multidimensional array  ConcatenateDimension=2
  Matrix Concatenate8 : Concatenate  NumInputs=3  Mode=Multidimensional array
  Matrix Concatenate9 : Concatenate  Mode=Multidimensional array  ConcatenateDimension=2
  Multiply{,1..5} (6 alike) : Gain  Gain=-1
  H : Outport
  wires:
  Matrix Concatenate10/1 -> H/1
  Matrix Concatenate4/1 -> Matrix Concatenate10/1
  [mat_xb] -> Matrix Concatenate9/1
  Matrix Concatenate9/1 -> Matrix Concatenate10/2
  3x3 0 matrix1/1 -> Matrix Concatenate9/2
  [row3bb] -> Matrix Concatenate8/3
  [row2bb] -> Matrix Concatenate8/2
  Matrix Concatenate8/1 -> [mat_xb]
  [row1bb] -> Matrix Concatenate8/1
  Matrix Concatenate6/1 -> [row2bb]
  [bb2] -> Multiply5/1
  [bb3] -> Matrix Concatenate6/1
  [bb3] -> Multiply3/1
  [bb2] -> Matrix Concatenate5/3
  Constant6/1 -> Matrix Concatenate7/3
  Matrix Concatenate7/1 -> [row3bb]
  [bb1] -> Multiply4/1
  Matrix Concatenate5/1 -> [row1bb]
  Multiply4/1 -> Matrix Concatenate6/3
  Constant5/1 -> Matrix Concatenate6/2
  Multiply3/1 -> Matrix Concatenate5/2
  Constant4/1 -> Matrix Concatenate5/1
  [bb1] -> Matrix Concatenate7/2
  Multiply5/1 -> Matrix Concatenate7/1
  Demux2/2 -> [bb2]
  Demux2/1 -> [bb1]
  bb_hat/1 -> Demux2/1
  Demux2/3 -> [bb3]
  rb_hat/1 -> Demux1/1
  Demux1/3 -> [rb3]
  [rb1] -> Matrix Concatenate2/2
  Constant2/1 -> Matrix Concatenate1/2
  Matrix Concatenate3/1 -> [mat_x]
  Demux1/1 -> [rb1]
  [row1rb] -> Matrix Concatenate3/1
  Constant1/1 -> Matrix Concatenate/1
  [row2rb] -> Matrix Concatenate3/2
  [rb3] -> Matrix Concatenate1/1
  [rb2] -> Matrix Concatenate/3
  [rb2] -> Multiply2/1
  3x3 0 matrix/1(0 3x3) -> Matrix Concatenate4/2
  Constant3/1 -> Matrix Concatenate2/3
  Multiply1/1 -> Matrix Concatenate1/3
  [rb3] -> Multiply/1
  [rb1] -> Multiply1/1
  Matrix Concatenate2/1 -> [row3rb]
  Matrix Concatenate/1 -> [row1rb]
  [row3rb] -> Matrix Concatenate3/3
  Multiply2/1 -> Matrix Concatenate2/1
  Demux1/2 -> [rb2]
  [mat_x] -> Matrix Concatenate4/1
  Multiply/1 -> Matrix Concatenate/2
  Matrix Concatenate1/1 -> [row2rb]

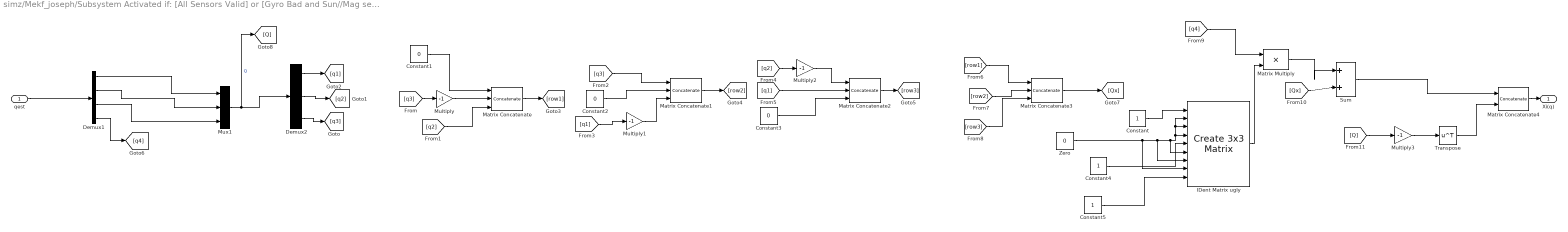
== system simz/Mekf_joseph/Subsystem Activated if: [All Sensors Valid] or [Gyro Bad and Sun//Mag sensors Valid]/Kalman Gain/Makes Xi(q) Matrix ==
  qest : Inport
  Constant : Constant
  Constant1 : Constant  Value=0
  Constant2 : Constant  Value=0
  Constant3 : Constant  Value=0
  Constant4 : Constant
  Constant5 : Constant
  Demux1 : Demux
  Demux2 : Demux  Outputs=3
  IDent Matrix ugly : sharedutil/Create 3x3 Matrix  aMode=aMode
  Matrix Concatenate : Concatenate  NumInputs=3  Mode=Multidimensional array  ConcatenateDimension=2
  Matrix Concatenate1 : Concatenate  NumInputs=3  Mode=Multidimensional array  ConcatenateDimension=2
  Matrix Concatenate2 : Concatenate  NumInputs=3  Mode=Multidimensional array  ConcatenateDimension=2
  Matrix Concatenate3 : Concatenate  NumInputs=3  Mode=Multidimensional array
  Matrix Concatenate4 : Concatenate  Mode=Multidimensional array
  Matrix Multiply : Product  Inputs=**
  Multiply{,1..3} (4 alike) : Gain  Gain=-1
  Mux1 : Mux  Inputs=3
  Sum : Sum  Inputs=|++
  Transpose : Math  Operator=transpose  SaturateOnIntegerOverflow=on
  Zero : Constant  Value=0  OutDataTypeStr=Inherit: Inherit via back propagation
  Xi(q) : Outport
  wires:
  Zero/1 -> IDent Matrix ugly/2, IDent Matrix ugly/3, IDent Matrix ugly/4, IDent Matrix ugly/6, IDent Matrix ugly/7, IDent Matrix ugly/8
  Constant4/1 -> IDent Matrix ugly/5
  Constant5/1 -> IDent Matrix ugly/9
  Constant/1 -> IDent Matrix ugly/1
  Matrix Concatenate4/1 -> Xi(q)/1
  Multiply1/1 -> Matrix Concatenate1/3
  [q1] -> Multiply1/1
  Constant3/1 -> Matrix Concatenate2/3
  Demux2/3 -> [q3]
  Matrix Concatenate/1 -> [row1]
  [q3] -> Multiply/1
  IDent Matrix ugly/1 -> Matrix Multiply/2
  Transpose/1 -> Matrix Concatenate4/2
  Demux2/1 -> [q1]
  [Q] -> Multiply3/1
  [row1] -> Matrix Concatenate3/1
  Multiply/1 -> Matrix Concatenate/2
  [Qx] -> Sum/2
  Matrix Concatenate2/1 -> [row3]
  Demux1/3 -> Mux1/3
  Demux1/1 -> Mux1/1
  [row2] -> Matrix Concatenate3/2
  Demux1/4 -> [q4]
  [q2] -> Multiply2/1
  Sum/1 -> Matrix Concatenate4/1
  Demux2/2 -> [q2]
  [q3] -> Matrix Concatenate1/1
  [q4] -> Matrix Multiply/1
  Multiply3/1 -> Transpose/1
  qest/1 -> Demux1/1
  [row3] -> Matrix Concatenate3/3
  Demux1/2 -> Mux1/2
  Constant2/1 -> Matrix Concatenate1/2
  Mux1/1 -> [Q], Demux2/1  "Q"
  [q2] -> Matrix Concatenate/3
  Matrix Concatenate3/1 -> [Qx]
  Constant1/1 -> Matrix Concatenate/1
  Matrix Concatenate1/1 -> [row2]
  Matrix Multiply/1 -> Sum/1
  [q1] -> Matrix Concatenate2/2
  Multiply2/1 -> Matrix Concatenate2/1

== system simz/Mekf_joseph/Subsystem Activated if: [All Sensors Valid] or [Gyro Bad and Sun//Mag sensors Valid]/TIME PROPAGATION of Q_EST, COVARIANCE/Psi ==
  In1 : Inport
  In2 : Inport  Port=2
  om_mags : Inport  Port=3
  om_magss : Inport  Port=4
  omega_vec : Inport  Port=5
  Divide : Product  Inputs=***
  Divide1 : Product  Inputs=**/
  Sin : Trigonometry
  Psi : Outport
  wires:
  om_magss/1 -> Divide1/3
  omega_vec/1 -> Divide1/2
  In2/1 -> Divide/2
  Sin/1 -> Divide1/1  "sin(om_mag*0.5*del_t)"
  om_mags/1 -> Divide/3
  Divide1/1 -> Psi/1  "Psi"
  Divide/1 -> Sin/1  "om_mag times0.5*del_t"
  In1/1 -> Divide/1

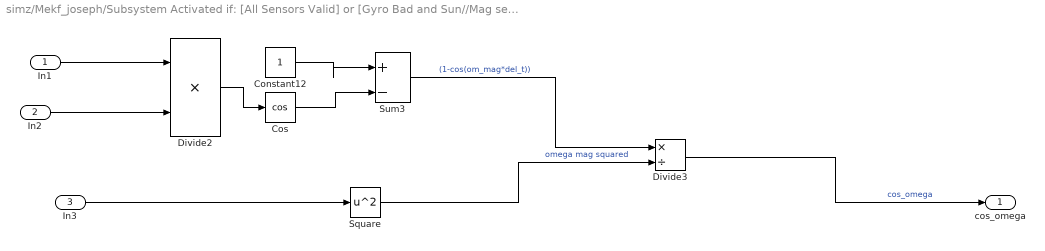
== system simz/Mekf_joseph/Subsystem Activated if: [All Sensors Valid] or [Gyro Bad and Sun//Mag sensors Valid]/TIME PROPAGATION of Q_EST, COVARIANCE/cos_omega ==
  In1 : Inport
  In2 : Inport  Port=2
  In3 : Inport  Port=3
  Constant12 : Constant
  Cos : Trigonometry  Operator=cos
  Divide2 : Product  Inputs=**
  Divide3 : Product  Inputs=*/
  Square : Math  Operator=square  SaturateOnIntegerOverflow=on
  Sum3 : Sum  Inputs=|+-
  cos_omega : Outport
  wires:
  Sum3/1 -> Divide3/1  "(1-cos(om_mag*del_t))"
  In2/1 -> Divide2/2
  Cos/1 -> Sum3/2
  In1/1 -> Divide2/1
  Square/1 -> Divide3/2  "omega mag squared"
  Constant12/1 -> Sum3/1
  Divide3/1 -> cos_omega/1  "cos_omega"
  In3/1 -> Square/1
  Divide2/1 -> Cos/1

== system simz/Mekf_joseph/Subsystem Activated if: [Sun//Mag Sensor Invalid and Gyros are Valid] or [Gyro Invalid and Sun//Mag sensors Invalid]/TIME PROPAGATION of Q_EST, COVARIANCE1/Psi ==
  In1 : Inport
  In2 : Inport  Port=2
  om_mags : Inport  Port=3
  om_magss : Inport  Port=4
  omega_vec : Inport  Port=5
  Divide : Product  Inputs=***
  Divide1 : Product  Inputs=**/
  Sin : Trigonometry
  Psi : Outport
  wires:
  om_magss/1 -> Divide1/3
  omega_vec/1 -> Divide1/2
  In2/1 -> Divide/2
  Sin/1 -> Divide1/1  "sin(om_mag*0.5*del_t)"
  om_mags/1 -> Divide/3
  Divide1/1 -> Psi/1  "Psi"
  Divide/1 -> Sin/1  "om_mag times0.5*del_t"
  In1/1 -> Divide/1

== system simz/Mekf_joseph/Subsystem Activated if: [Sun//Mag Sensor Invalid and Gyros are Valid] or [Gyro Invalid and Sun//Mag sensors Invalid]/TIME PROPAGATION of Q_EST, COVARIANCE1/cos_omega ==
  In1 : Inport
  In2 : Inport  Port=2
  In3 : Inport  Port=3
  Constant12 : Constant
  Cos : Trigonometry  Operator=cos
  Divide2 : Product  Inputs=**
  Divide3 : Product  Inputs=*/
  Square : Math  Operator=square  SaturateOnIntegerOverflow=on
  Sum3 : Sum  Inputs=|+-
  cos_omega : Outport
  wires:
  Sum3/1 -> Divide3/1  "(1-cos(om_mag*del_t))"
  In2/1 -> Divide2/2
  Cos/1 -> Sum3/2
  In1/1 -> Divide2/1
  Square/1 -> Divide3/2  "omega mag squared"
  Constant12/1 -> Sum3/1
  Divide3/1 -> cos_omega/1  "cos_omega"
  In3/1 -> Square/1
  Divide2/1 -> Cos/1

== system simz/Mekf_joseph/Subsystem Activated if: [All Sensors Valid] or [Gyro Bad and Sun//Mag sensors Valid]/Kalman Gain/Create H matrix/3x3 0 matrix ==
  Create 3x3 Matrix : sharedutil/Create 3x3 Matrix  aMode=aMode
  Zero : Constant  Value=0  OutDataTypeStr=Inherit: Inherit via back propagation
  0 3x3 : Outport
  wires:
  Create 3x3 Matrix/1 -> 0 3x3/1
  Zero/1 -> Create 3x3 Matrix/4, Create 3x3 Matrix/3, Create 3x3 Matrix/2, Create 3x3 Matrix/5, Create 3x3 Matrix/1, Create 3x3 Matrix/6, Create 3x3 Matrix/7, Create 3x3 Matrix/8, Create 3x3 Matrix/9

== matlab function simz/Mekf_joseph/Subsystem Activated if: [All Sensors Valid] or [Gyro Bad and Sun//Mag sensors Valid]/Kalman Gain/kalman gain, P update ==
  data: R input; Pplus output size=[6,6]; Pminus input; H input; K output size=[6,6]
function [Pplus,K] = fcn113(R,Pminus,H)
K = Pminus*H'*inv(H*Pminus*H' + R);
        
        %%%Update
        Pplus = (eye(6)-K*H)*Pminus;
        
%         KHI = (K*H - eye(6));
%         Pplus= KHI*Pminus*KHI' + K*R*K';
%         Pplus = (eye(6)-K*H)*Pminus*(eye(6)-K*H)' + K*R*K';
end

== matlab function simz/Mekf_joseph/Subsystem Activated if: [All Sensors Valid] or [Gyro Bad and Sun//Mag sensors Valid]/TIME PROPAGATION of Q_EST, COVARIANCE/MATLAB Function7 ==
  data: Psi input; Psi_cross output
function Psi_cross = Psi_cross_matrix(Psi)
%#codegen

Psi_cross = [0 -Psi(3) Psi(2);Psi(3) 0 -Psi(1);-Psi(2) Psi(1) 0];

== matlab function simz/Mekf_joseph/Subsystem Activated if: [All Sensors Valid] or [Gyro Bad and Sun//Mag sensors Valid]/TIME PROPAGATION of Q_EST, COVARIANCE/MATLAB Function8 ==
  data: Psi_x input; Psi input; om_mag input; del_t input; Omega_omega output
function Omega_omega = omega_omega_matrix(Psi_x,Psi,om_mag,del_t)
%#codegen

 Omega_omega = [(cos(0.5*om_mag*del_t)*eye(3) - Psi_x), Psi; -Psi', cos(0.5*om_mag*del_t)];

== matlab function simz/Mekf_joseph/Subsystem Activated if: [All Sensors Valid] or [Gyro Bad and Sun//Mag sensors Valid]/TIME PROPAGATION of Q_EST, COVARIANCE/MATLAB Function10 ==
  data: dt input; om_mag input; omega_x input; Phi output
function Phi = Phi_disc(dt,om_mag,omega_x)
%#codegen

% State_Trans_matrix = [(eye(3)-omega_x*sin(om_mag*del_t)/om_mag + (omega_x^2)*cos_omega),omega_x*cos_omega-eye(3)*del_t-omega_x^2*(om_mag*del_t-sin(om_mag*del_t))/om_mag^3;
%             zeros(3,3),eye(3)];

w_n     = om_mag;
w_skew  = omega_x;

if( w_n < 1e-10 )
    Phi = [ eye(3)     -eye(3)*dt;
            zeros(3,3)  eye(3) ];
else
    Phi_11  = eye(3) - w_skew*(sin(w_n*dt)/w_n) + ...
                                        w_skew^2*(1 - cos(w_n*dt))/w_n^2;
    Phi_12  = w_skew*(1 - cos(w_n*dt))/w_n^2 - eye(3)*dt - ...
                                    w_skew^2*(w_n*dt - sin(w_n*dt))/w_n^3;
    Phi_21  = zeros(3,3);    
    Phi_22  = eye(3);    
    Phi     = [ Phi_11 Phi_12;
                Phi_21 Phi_22 ];
end

== matlab function simz/Mekf_joseph/Subsystem Activated if: [All Sensors Valid] or [Gyro Bad and Sun//Mag sensors Valid]/TIME PROPAGATION of Q_EST, COVARIANCE/MATLAB Function1 ==
  data: Phi_discrete input; P_plus input; Qg input; P_prop output size=[6,6]
function P_prop = P_kplus1(Phi_discrete,P_plus,Qg)
%#codegen
P_prop = Phi_discrete*P_plus*Phi_discrete' + Qg;

== matlab function simz/Mekf_joseph/Subsystem Activated if: [All Sensors Valid] or [Gyro Bad and Sun//Mag sensors Valid]/TIME PROPAGATION of Q_EST, COVARIANCE/MATLAB Function9 ==
  data: omega input; omega_cross_matrix output
function omega_cross_matrix = makes_omega_cross_matrix(omega)

omega_cross_matrix = [0 -omega(3) omega(2);omega(3) 0 -omega(1);-omega(2) omega(1) 0];

== matlab function simz/Mekf_joseph/Subsystem Activated if: [All Sensors Valid] or [Gyro Bad and Sun//Mag sensors Valid]/Kalman Gain/MATLAB Function ==
  data: qe input; XI output
function XI = fcn(qe)
%#codegen

XI = [ -qe(2) -qe(3) -qe(4);
        qe(1) -qe(4)  qe(3);
        qe(4)  qe(1) -qe(2);
       -qe(3)  qe(2)  qe(1) ];

== matlab function simz/Mekf_joseph/Subsystem Activated if: [All Sensors Valid] or [Gyro Bad and Sun//Mag sensors Valid]/TIME PROPAGATION of Q_EST, COVARIANCE/MATLAB Function ==
  data: omega_est input; om_mag output
function om_mag = om2_norm(omega_est)

om_mag = norm(omega_est);

== matlab function simz/Mekf_joseph/Subsystem Activated if: [All Sensors Valid] or [Gyro Bad and Sun//Mag sensors Valid]/TIME PROPAGATION of Q_EST, COVARIANCE/MATLAB Function2 ==
  data: u input; om_mag output
function om_mag = norm_check1(u)
%#codegen
if u == 0
    om_mag = 10^-10;
else
    om_mag = u;
end
end

== matlab function simz/Mekf_joseph/Subsystem Activated if: [All Sensors Valid] or [Gyro Bad and Sun//Mag sensors Valid]/Kalman Gain/MATLAB Function1 ==
  data: rb_hat input; H output; bb_hat input
function H  = fcn1133(rb_hat,bb_hat)

           mat = rb_hat;
            mat_x = [0 -mat(3) mat(2);mat(3) 0 -mat(1);-mat(2) mat(1) 0]; %cross product matrix of q
        mat1 = bb_hat;
            mat_x1 = [0 -mat1(3) mat1(2);mat1(3) 0 -mat1(1);-mat1(2) mat1(1) 0];
%         Ri_x = [0 -Ri(3) Ri(2);Ri(3) 0 -Ri(1);-Ri(2) Ri(1) 0];
%         Bb_x = [0 -Bb(3) Bb(2);Bb(3) 0 -Bb(1);-Bb(2) Bb(1) 0];
%%%%% Calcualte Kalman Gain
        H = [mat_x, zeros(3,3);mat_x1,zeros(3,3)];
end

== matlab function simz/Mekf_joseph/Subsystem Activated if: [All Sensors Valid] or [Gyro Bad and Sun//Mag sensors Valid]/MEASUREMENT UPDATE TO q /MATLAB Function ==
  data: qe input; qep_norm output size=[4]
function qep_norm = norm(qe)
%#codegen

qep_norm = 1/(norm(qe))*qe;

== matlab function simz/Mekf_joseph/Subsystem Activated if: [All Sensors Valid] or [Gyro Bad and Sun//Mag sensors Valid]/Kalman Gain/MATLAB Function3 ==
  data: qe input; H output size=[6,6]; s2c_sun_eci_unit input; mag_eci_unit input; s_hat output size=[3,1]; b_hat output size=[3,1]
function [H,s_hat,b_hat] = fcn(qe,s2c_sun_eci_unit,mag_eci_unit)
%#codegen
    q0 = qe(1);
qv = qe(2:4);
dcm = (2*q0^2-1)*eye(3) + 2*(qv*qv') - 2*q0*skew(qv);
   s_hat = dcm*s2c_sun_eci_unit;
            s_hat_x = [0 -s_hat(3) s_hat(2);s_hat(3) 0 -s_hat(1);-s_hat(2) s_hat(1) 0]; %cross product s_hatrix of q
        b_hat = dcm*mag_eci_unit;
            b_hat_x = [0 -b_hat(3) b_hat(2);b_hat(3) 0 -b_hat(1);-b_hat(2) b_hat(1) 0];

        H = [s_hat_x, zeros(3,3);b_hat_x,zeros(3,3)];
end

== matlab function simz/Mekf_joseph/Subsystem Activated if: [Sun//Mag Sensor Invalid and Gyros are Valid] or [Gyro Invalid and Sun//Mag sensors Invalid]/TIME PROPAGATION of Q_EST, COVARIANCE1/MATLAB Function ==
  data: omega_est input; om_mag output
function om_mag = om2_norm(omega_est)

om_mag = norm(omega_est);

== matlab function simz/Mekf_joseph/Subsystem Activated if: [Sun//Mag Sensor Invalid and Gyros are Valid] or [Gyro Invalid and Sun//Mag sensors Invalid]/TIME PROPAGATION of Q_EST, COVARIANCE1/MATLAB Function1 ==
  data: Phi_discrete input; P_plus input; Qg input; P_prop output size=[6,6]
function P_prop = P_kplus1(Phi_discrete,P_plus,Qg)
%#codegen
P_prop = Phi_discrete*P_plus*Phi_discrete' + Qg;

== matlab function simz/Mekf_joseph/Subsystem Activated if: [Sun//Mag Sensor Invalid and Gyros are Valid] or [Gyro Invalid and Sun//Mag sensors Invalid]/TIME PROPAGATION of Q_EST, COVARIANCE1/MATLAB Function10 ==
  data: dt input; om_mag input; omega_x input; Phi output
function Phi = Phi_disc(dt,om_mag,omega_x)
%#codegen

% State_Trans_matrix = [(eye(3)-omega_x*sin(om_mag*del_t)/om_mag + (omega_x^2)*cos_omega),omega_x*cos_omega-eye(3)*del_t-omega_x^2*(om_mag*del_t-sin(om_mag*del_t))/om_mag^3;
%             zeros(3,3),eye(3)];

w_n     = om_mag;
w_skew  = omega_x;

if( w_n < 1e-10 )
    Phi = [ eye(3)     -eye(3)*dt;
            zeros(3,3)  eye(3) ];
else
    Phi_11  = eye(3) - w_skew*(sin(w_n*dt)/w_n) + ...
                                        w_skew^2*(1 - cos(w_n*dt))/w_n^2;
    Phi_12  = w_skew*(1 - cos(w_n*dt))/w_n^2 - eye(3)*dt - ...
                                    w_skew^2*(w_n*dt - sin(w_n*dt))/w_n^3;
    Phi_21  = zeros(3,3);    
    Phi_22  = eye(3);    
    Phi     = [ Phi_11 Phi_12;
                Phi_21 Phi_22 ];
end

== matlab function simz/Mekf_joseph/Subsystem Activated if: [Sun//Mag Sensor Invalid and Gyros are Valid] or [Gyro Invalid and Sun//Mag sensors Invalid]/TIME PROPAGATION of Q_EST, COVARIANCE1/MATLAB Function2 ==
  data: u input; om_mag output
function om_mag = norm_check1(u)
%#codegen
if u == 0
    om_mag = 10^-10;
else
    om_mag = u;
end
end

== matlab function simz/Mekf_joseph/Subsystem Activated if: [Sun//Mag Sensor Invalid and Gyros are Valid] or [Gyro Invalid and Sun//Mag sensors Invalid]/TIME PROPAGATION of Q_EST, COVARIANCE1/MATLAB Function7 ==
  data: Psi input; Psi_cross output
function Psi_cross = Psi_cross_matrix(Psi)
%#codegen

Psi_cross = [0 -Psi(3) Psi(2);Psi(3) 0 -Psi(1);-Psi(2) Psi(1) 0];

== matlab function simz/Mekf_joseph/Subsystem Activated if: [Sun//Mag Sensor Invalid and Gyros are Valid] or [Gyro Invalid and Sun//Mag sensors Invalid]/TIME PROPAGATION of Q_EST, COVARIANCE1/MATLAB Function8 ==
  data: Psi_x input; Psi input; om_mag input; del_t input; Omega_omega output
function Omega_omega = omega_omega_matrix(Psi_x,Psi,om_mag,del_t)
%#codegen

 Omega_omega = [(cos(0.5*om_mag*del_t)*eye(3) - Psi_x), Psi; -Psi', cos(0.5*om_mag*del_t)];

== matlab function simz/Mekf_joseph/Subsystem Activated if: [Sun//Mag Sensor Invalid and Gyros are Valid] or [Gyro Invalid and Sun//Mag sensors Invalid]/TIME PROPAGATION of Q_EST, COVARIANCE1/MATLAB Function9 ==
  data: omega input; omega_cross_matrix output
function omega_cross_matrix = makes_omega_cross_matrix(omega)

omega_cross_matrix = [0 -omega(3) omega(2);omega(3) 0 -omega(1);-omega(2) omega(1) 0];
